simulink model "ACE_Exh_sys_new"  (R2016a)
settings: Solver=VariableStepAuto  SolverMode=SingleTasking  StartTime=0.0  StopTime=5  RelTol=0.1
libraries: simulink x1
settings Model: Creator=Devashree  LastModifiedBy=Devashree
settings SolverCC: AlgebraicLoopSolver=LineSearch
settings DebuggingCC: SFUnexpectedBacktrackingDiag=error  SFNoUnconditionalDefaultTransitionDiag=error
settings GRTTargetCC: TargetLangStandard=C99 (ISO)  GeneratePreprocessorConditionals=Use local settings
settings ConfigComp: CovMetricSettings=dwe  CovHtmlReporting=off  CovSaveCumulativeToWorkspaceVar=off  CovSaveSingleToWorkspaceVar=off  CovExternalEMLEnable=on

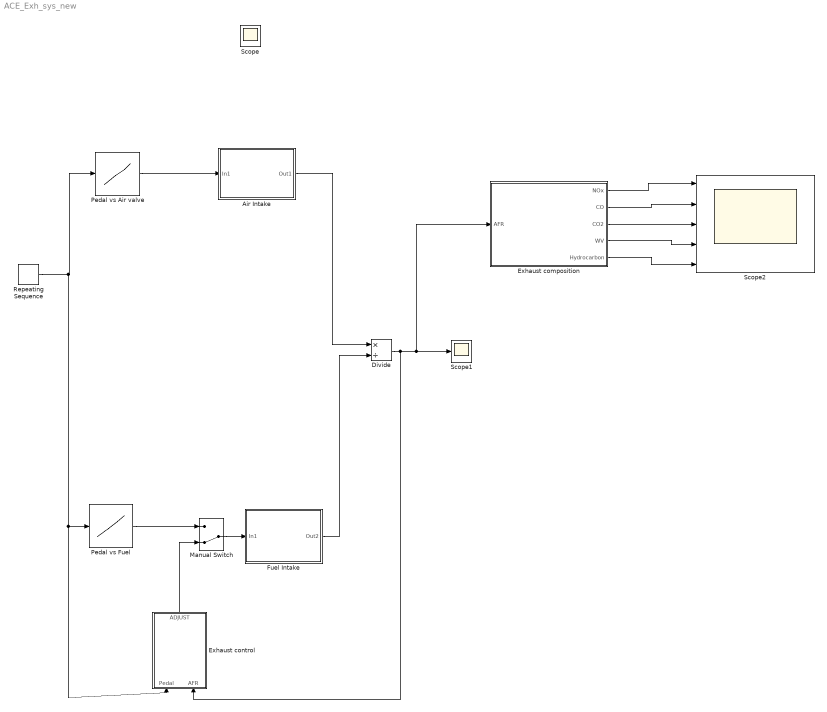
== system ACE_Exh_sys_new ==
  Air Intake : Subsystem
  Divide : Product  Inputs=*/
  Exhaust composition : Subsystem
  Exhaust control : Subsystem
  Fuel Intake : Subsystem
  Manual Switch : ManualSwitch  CurrentSetting=0
  Pedal vs Air valve : Lookup_n-D  NumberOfTableDimensions=1  BreakpointsForDimension1=[0.1 0.5 1 2 5 7 10]  Table=|  InternalRulePriority=Speed  RndMeth=Simplest  InputSameDT=on
      | [1
      | 15
      | 10
      | 20
      | 50
      | 70
      | 100]
  Pedal vs Fuel : Lookup_n-D  NumberOfTableDimensions=1  BreakpointsForDimension1=[0.1 0.5 1 2 5 7 10]  BreakpointsForDimension1FirstPoint=5.4517133956386  Table=|  InternalRulePriority=Speed  RndMeth=Simplest  InputSameDT=on
      | [0.48
      | 15
      | 20
      | 18
      | 50
      | 65
      | 100]
  Repeating Sequence : simulink/Sources/Repeating Sequence  rep_seq_t=|  rep_seq_y=|
      rep_seq_t=|
      | [0
      | 0.5
      | 1
      | 1.5
      | 2
      | 2.5
      | 3
      | 3.5
      | 4
      | 4.5
      | 5]
      rep_seq_y=|
      | [1
      | 5
      | 2
      | 4
      | 7
      | 10
      | 10
      | 5
      | 2
      | 4
      | 7]
  Scope1 : Scope
  Scope2 : Scope  NumInputPorts=5
  Scope : Scope
  wires:
  Air Intake/1(Out1) -> Divide/1
  Pedal vs Fuel/1 -> Manual Switch/1
  Repeating Sequence/1 -> Pedal vs Fuel/1, Exhaust control/1(Pedal), Pedal vs Air valve/1
  Manual Switch/1 -> Fuel Intake/1(In1)
  Fuel Intake/1(Out2) -> Divide/2
  Divide/1 -> Exhaust composition/1(AFR), Scope1/1, Exhaust control/2(AFR)
  Exhaust composition/1(NOx) -> Scope2/1
  Exhaust composition/2(CO) -> Scope2/2
  Exhaust composition/3(CO2) -> Scope2/3
  Exhaust composition/4(WV) -> Scope2/4
  Exhaust composition/5(Hydrocarbon) -> Scope2/5
  Exhaust control/1(ADJUST) -> Manual Switch/2
  Pedal vs Air valve/1 -> Air Intake/1(In1)

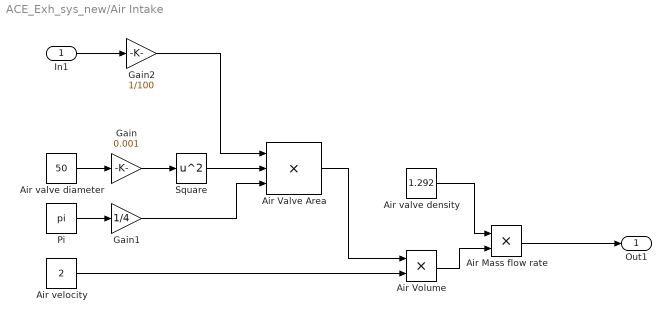
== system ACE_Exh_sys_new/Air Intake ==
  In1 : Inport
  Air Mass flow rate : Product
  Air Valve Area : Product  Inputs=3
  Air Volume : Product
  Air valve density : Constant  Value=1.292
  Air valve diameter : Constant  Value=50
  Air velocity : Constant  Value=2
  Gain : Gain  Gain=0.001
  Gain1 : Gain  Gain=1/4
  Gain2 : Gain  Gain=1/100
  Pi : Constant  Value=pi
  Square : Math  Operator=square  SaturateOnIntegerOverflow=on
  Out1 : Outport
  wires:
  Gain/1 -> Square/1
  Pi/1 -> Gain1/1
  Air Valve Area/1 -> Air Volume/1
  Air velocity/1 -> Air Volume/2
  Air valve diameter/1 -> Gain/1
  Air Volume/1 -> Air Mass flow rate/2
  Air valve density/1 -> Air Mass flow rate/1
  Air Mass flow rate/1 -> Out1/1
  Square/1 -> Air Valve Area/2
  Gain1/1 -> Air Valve Area/3
  In1/1 -> Gain2/1
  Gain2/1 -> Air Valve Area/1

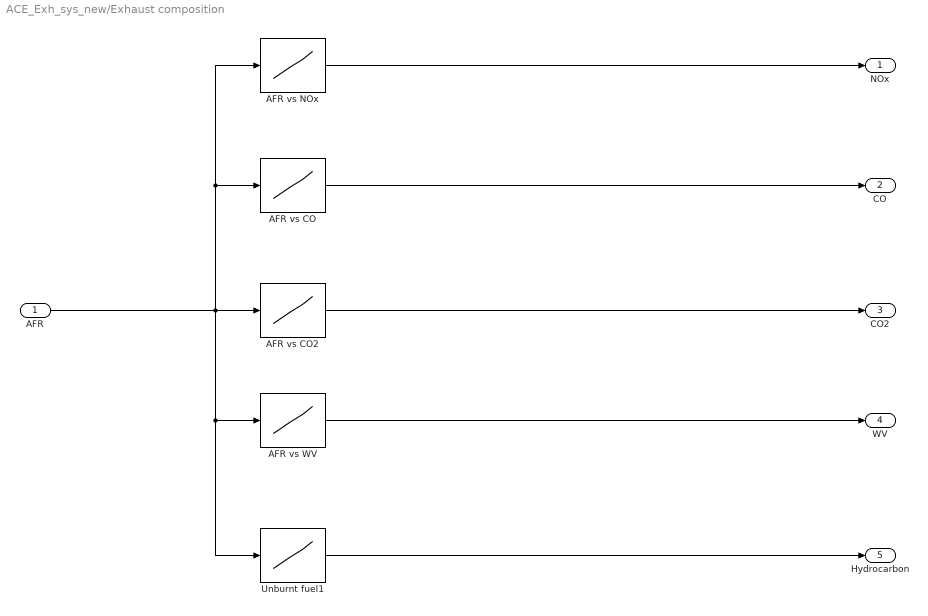
== system ACE_Exh_sys_new/Exhaust composition ==
  AFR : Inport
  AFR vs CO : Lookup_n-D  NumberOfTableDimensions=1  BreakpointsForDimension1=[10 14.5 14.6 14.7 14.8 15 15.5 18]  BreakpointsForDimension1FirstPoint=5.4517133956386  Table=[12 8 4 0.1 0.1 0.05 0.03 0.015]  InternalRulePriority=Speed  RndMeth=Simplest  InputSameDT=on
  AFR vs CO2 : Lookup_n-D  NumberOfTableDimensions=1  BreakpointsForDimension1=[10 14.5 14.6 14.7 14.8 15 15.5 18]  BreakpointsForDimension1FirstPoint=5.4517133956386  Table=[13 13 13.5 14 14 15 15 16]  InternalRulePriority=Speed  RndMeth=Simplest  InputSameDT=on
  "AFR vs NOx " : Lookup_n-D  NumberOfTableDimensions=1  BreakpointsForDimension1=[10 14.5 14.6 14.7 14.8 15 15.5 18]  BreakpointsForDimension1FirstPoint=5.4517133956386  Table=[1 2.5 5 10 20 30 50 65]  InternalRulePriority=Speed  RndMeth=Simplest  InputSameDT=on
  AFR vs WV : Lookup_n-D  NumberOfTableDimensions=1  BreakpointsForDimension1=[10 14.5 14.6 14.7 14.8 15 15.5 18]  BreakpointsForDimension1FirstPoint=5.4517133956386  Table=[12 12 12.5 13 13 13 14 14]  InternalRulePriority=Speed  RndMeth=Simplest  InputSameDT=on
  Unburnt fuel1 : Lookup_n-D  NumberOfTableDimensions=1  BreakpointsForDimension1=[10 14.1 14.5 14.6 14.7 14.8 15 15.5 18]  BreakpointsForDimension1FirstPoint=5.4517133956386  Table=[6 3 2 1.5 0 0 0 0 0]  InternalRulePriority=Speed  RndMeth=Simplest  InputSameDT=on
  NOx : Outport
  CO : Outport  Port=2
  CO2 : Outport  Port=3
  WV : Outport  Port=4
  Hydrocarbon : Outport  Port=5
  wires:
  AFR/1 -> "AFR vs NOx "/1, AFR vs CO/1, AFR vs CO2/1, Unburnt fuel1/1, AFR vs WV/1
  "AFR vs NOx "/1 -> NOx/1
  AFR vs CO/1 -> CO/1
  AFR vs CO2/1 -> CO2/1
  AFR vs WV/1 -> WV/1
  Unburnt fuel1/1 -> Hydrocarbon/1

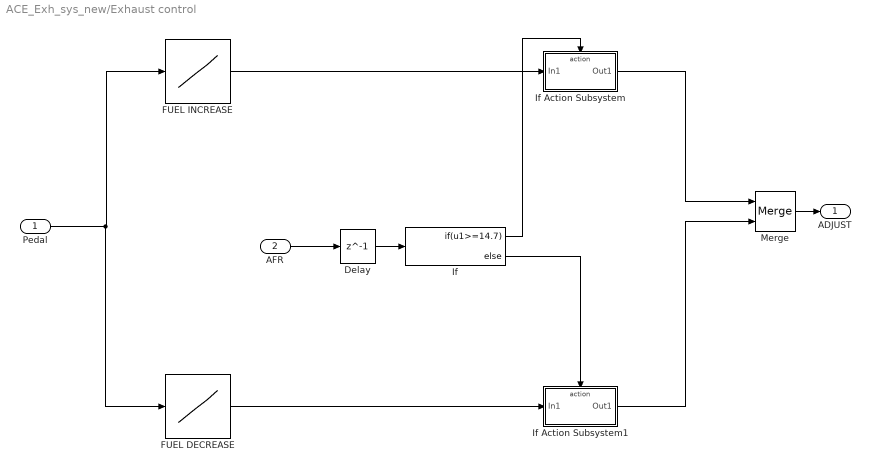
== system ACE_Exh_sys_new/Exhaust control ==
  Pedal : Inport
  AFR : Inport  Port=2
  Delay : Delay  DelayLength=1  InitialCondition=0
  FUEL DECREASE : Lookup_n-D  NumberOfTableDimensions=1  BreakpointsForDimension1=[0.1 0.5 1 2 5 7 10]  BreakpointsForDimension2=[1 7 10 14.7 16 20 40]  Table=|  InternalRulePriority=Speed  RndMeth=Simplest  InputSameDT=on
      | [0.5
      | 15
      | 20
      | 20
      | 50
      | 70
      | 100]
  FUEL INCREASE : Lookup_n-D  NumberOfTableDimensions=1  BreakpointsForDimension1=[0.1 0.5 1 2 5 7 10]  Table=|  InternalRulePriority=Speed  RndMeth=Simplest  InputSameDT=on
      | [0.5
      | 15
      | 20
      | 20
      | 50
      | 70
      | 100]
  If : If  IfExpression=u1>=14.7
  If Action Subsystem : Subsystem  TreatAsAtomicUnit=on
  If Action Subsystem1 : Subsystem  TreatAsAtomicUnit=on
  Merge : Merge
  ADJUST : Outport
  wires:
  AFR/1 -> Delay/1
  If/1 -> If Action Subsystem/Action
  Delay/1 -> If/1
  If/2 -> If Action Subsystem1/Action
  FUEL INCREASE/1 -> If Action Subsystem/1(In1)
  Pedal/1 -> FUEL DECREASE/1, FUEL INCREASE/1
  FUEL DECREASE/1 -> If Action Subsystem1/1(In1)
  Merge/1 -> ADJUST/1
  If Action Subsystem/1(Out1) -> Merge/1
  If Action Subsystem1/1(Out1) -> Merge/2

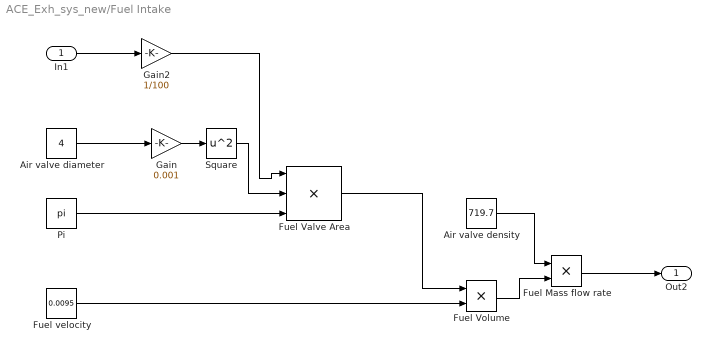
== system ACE_Exh_sys_new/Fuel Intake ==
  In1 : Inport
  Air valve density : Constant  Value=719.7
  Air valve diameter : Constant  Value=4
  Fuel Mass flow rate : Product
  Fuel Valve Area : Product  Inputs=3
  Fuel Volume : Product
  Fuel velocity : Constant  Value=0.0095
  Gain : Gain  Gain=0.001
  Gain2 : Gain  Gain=1/100
  Pi : Constant  Value=pi
  Square : Math  Operator=square  SaturateOnIntegerOverflow=on
  Out2 : Outport
  wires:
  Gain/1 -> Square/1
  Fuel velocity/1 -> Fuel Volume/2
  Fuel Volume/1 -> Fuel Mass flow rate/2
  Air valve density/1 -> Fuel Mass flow rate/1
  Fuel Valve Area/1 -> Fuel Volume/1
  Fuel Mass flow rate/1 -> Out2/1
  Air valve diameter/1 -> Gain/1
  Gain2/1 -> Fuel Valve Area/1
  In1/1 -> Gain2/1
  Square/1 -> Fuel Valve Area/2
  Pi/1 -> Fuel Valve Area/3

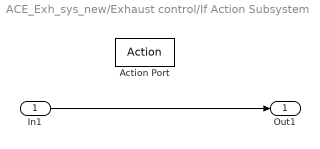
== system ACE_Exh_sys_new/Exhaust control/If Action Subsystem ==
  In1 : Inport
  Action Port : ActionPort  ActionType=then
  Out1 : Outport
  wires:
  In1/1 -> Out1/1

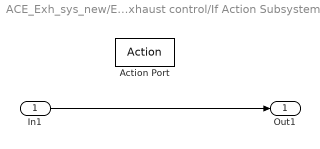
== system ACE_Exh_sys_new/Exhaust control/If Action Subsystem1 ==
  In1 : Inport
  Action Port : ActionPort  ActionType=else
  Out1 : Outport
  wires:
  In1/1 -> Out1/1
